simulink model "pendulum_continuous"  (R2024b)
settings: Solver=VariableStepAuto  StartTime=0.0  StopTime=100  RelTol=1e-3
settings Model: Creator=Botló  LastModifiedBy=Botló

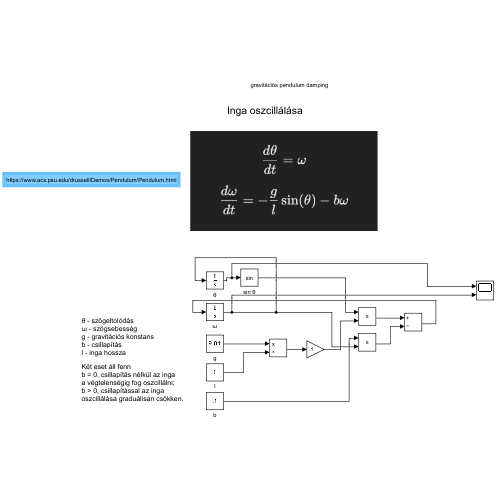
[thumbnail: Simulink's stored preview of the top-level diagram]
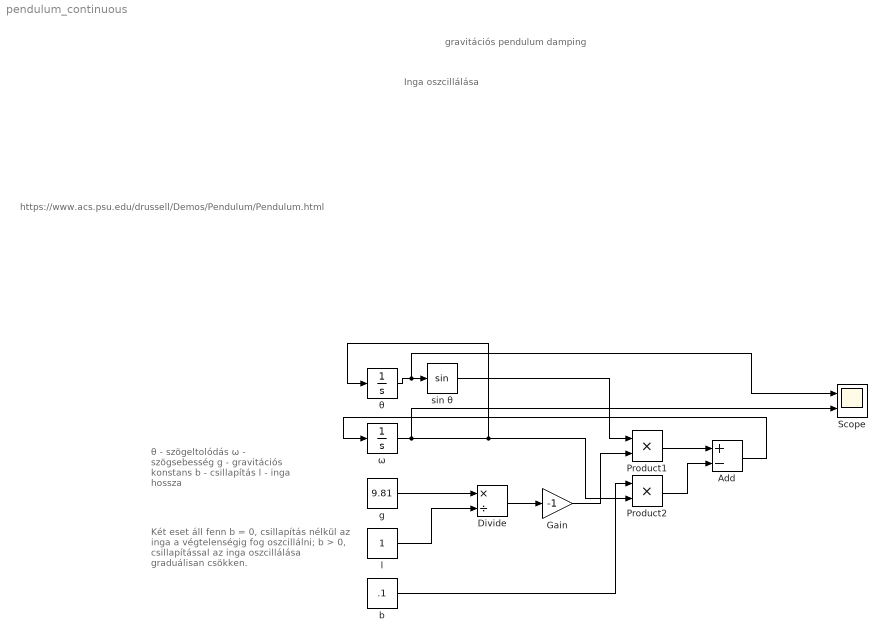
== system pendulum_continuous ==
  note: https://www.acs.psu.edu/drussell/Demos/Pendulum/Pendulum.html
  note: Két eset áll fenn
      | b = 0, csillapítás nélkül az inga
      | a végtelenségig fog oszcillálni;
      | b > 0, csillapítással az inga
      | oszcillálása graduálisan csökken.
  note: Inga oszcillálása
  note: θ - szögeltolódás
      | ω - szögsebesség
      | g - gravitációs konstans
      | b - csillapítás
      | l - inga hossza
  note: gravitációs pendulum damping
  Add : Sum  Inputs=+-
  Divide : Product  Inputs=*/
  Gain : Gain  Gain=-1
  Product1 : Product
  Product2 : Product
  Scope : Scope  NumInputPorts=2
  b : Constant  Value=.1
  g : Constant  Value=9.81
  l : Constant
  sin θ : Trigonometry
  θ : Integrator  InitialCondition=0.1
  ω : Integrator
  wires:
  g/1 -> Divide/1
  l/1 -> Divide/2
  sin θ/1 -> Product1/1
  Gain/1 -> Product1/2
  Product1/1 -> Add/1
  Product2/1 -> Add/2
  b/1 -> Product2/1
  ω/1 -> θ/1, Product2/2, Scope/2
  Add/1 -> ω/1
  Divide/1 -> Gain/1
  θ/1 -> Scope/1, sin θ/1
